simulink model "four_module_inverter_9_level_MCI"  (R2025a)
settings: Solver=VariableStepAuto  StartTime=0.0  StopTime=1  RelTol=1e-3
undefined symbols (not defined in the file): Ion, Lithium
libraries: spsIGBTDiodeLib x16, simulink x8, spsCurrentMeasurementLib x6, spsBreakerLib x4, spsBatteryLib x4, spsVoltageMeasurementLib x3, spsRMSLib x1, spsTHDLib x1, sps_lib x1
settings Model: Creator=mugun  LastModifiedBy=mugun
settings DataIOCC: SaveFormat=StructureWithTime  LoggingToFile=on

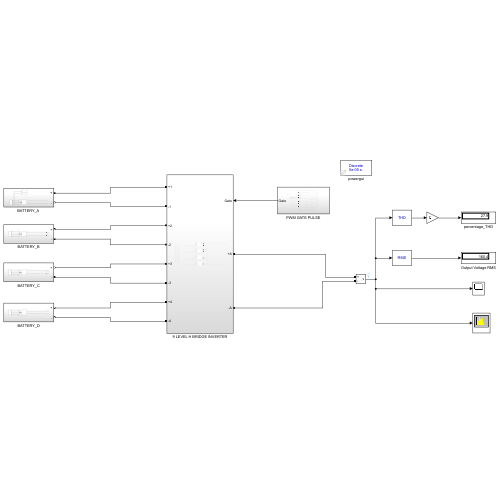
[thumbnail: Simulink's stored preview of the top-level diagram]
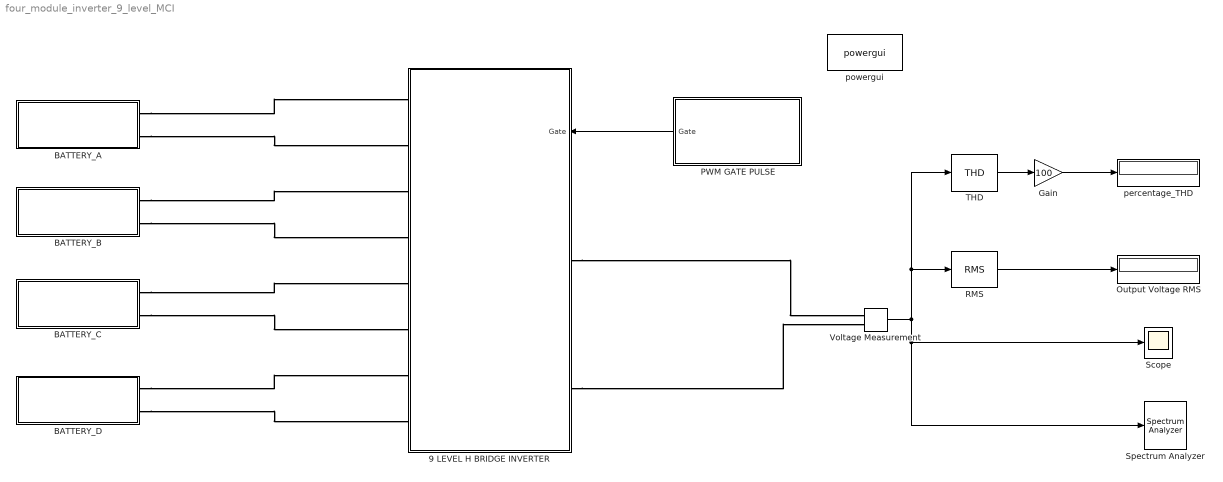
== system four_module_inverter_9_level_MCI ==
  9 LEVEL H BRIDGE INVERTER : Subsystem
      settings: PortSchema="{\"entries\":[{\"content\":{\"sides\":[{\"content\":{\"connectorIds\":[\"LConn1\",\"LConn2\",\"LConn3\",\"LConn4\",\"LConn5\",\"LConn6\",\"LConn7\",\"LConn8\"]},\"type\":\"ConnectorPlacement.EquallySpacedRectSide\",\"uuid\":\"a99ba5a4-868b-4ca9-ae89-158e30df76de\"},{\"content\":{\"connectorIds\":[\"In1\",\"RConn1\",\"RConn2\"],\"side\":\"RIGHT\"},\"type\":\"ConnectorPlacement.EquallySpacedRectSide\",\"uuid\":\"907b6b32-6b28-4f9b-aa63-058c17a50e82\"},{\"content\":{\"side\":\"TOP\"},\"type\":\"ConnectorPlacement.EquallySpacedRectSide\",\"uuid\":\"64bd340d-5502-4b77-92cb-0ed146f38aa8\"}]},\"type\":\"ConnectorPlacement.EquallySpacedConnector\",\"uuid\":\"1fa2cca1-805b-4996-9e9c-123ddddb2b33\"}],\"packageUris\":[\"http://schema.mathworks.com/mf0/Connector/R2020b\"],\"version\":\"1.0\"}"
  "BATTERY_A " : Subsystem
  BATTERY_B : Subsystem
  BATTERY_C : Subsystem
  BATTERY_D : Subsystem
  Gain : Gain  Gain=100
  Output Voltage RMS : Display
  PWM GATE PULSE : Subsystem
  RMS : spsRMSLib/RMS  TrueRMS=on  Freq=60  RMSInit=120  Ts=0
  Scope : Scope
      settings: ActiveDisplayYMinimum=-302.46098091950148  ActiveDisplayYMaximum=306.52866411781525  DataLoggingVariableName=MCI_nine
  Spectrum Analyzer : SpectrumAnalyzer  WindowPosition=[1.000000,49.000000,1536.000000,793.000000,]  ScopeFrameLocation=window  Method=Welch  PlotAsTwoSidedSpectrum=off  AveragingMethod=Exponential  MaximizeAxes=Off  YLimits=[-0.4051 87.1177]  SelectedToolstripTab=spectrumAnalyzerToolstrip.measurementsTab
  THD : spsTHDLib/THD  Freq=60  Ts=0
  Voltage Measurement : spsVoltageMeasurementLib/Voltage Measurement  PhasorSimulation=off  OutputType=Complex  PSBequivalent=0
  percentage_THD : Display
  powergui : sps_lib/powergui  Priority=1  SimulationMode=Discrete  SampleTime=50e-6  frequency=60  Iterations=50  frequencyindice=0  Pbase=100e6  ErrMax=1e-4  UnitsV=kV  UnitsW=MW  buscounter=0  FunctionMessages=off  echomessages=off  EnableUseOfTLC=off  CurrentSourceSwitches=off  DisableSnubberDevices=off  DisableRonSwitches=off  DisableVfSwitches=off  DisplayEquations=off  AutomaticDiscreteSolvers=off  SolverType=Tustin/Backward Euler (TBE)  Interpol=off  ExternalGateDelay=off  methode=off  Ts=100  x0status=blocks  SPID=on  SwTol=0  HookPort=off  NonlinearTolerance=1e-4  nMaxIteration=100  ContinueOnMaxIteration=off  RestoreLinks=warning  ResistiveCurrentMeasurement=off  Frange=[0:2:500]  Ylog=off  Xlog=on  ShowGrid=off  save=off  variable=ZData  structure=0  ZoomFFT=off  StartTime=0.0  cycles=1  DisplayStyle=1  fundamental=60  FreqAxis=off  MaxFrequency=1000  frequencyindicesteady=1  RmsSteady=1  display=off
  wires:
  PWM GATE PULSE/1(Gate) -> 9 LEVEL H BRIDGE INVERTER/1(Gate)
  Voltage Measurement/1 -> Scope/1, Spectrum Analyzer/1, THD/1, RMS/1
  RMS/1 -> Output Voltage RMS/1
  THD/1 -> Gain/1
  Gain/1 -> percentage_THD/1
  connections:
  BATTERY_D/LConn1 -- 9 LEVEL H BRIDGE INVERTER/LConn7
  BATTERY_C/LConn1 -- 9 LEVEL H BRIDGE INVERTER/LConn5
  BATTERY_D/LConn2 -- 9 LEVEL H BRIDGE INVERTER/LConn8
  BATTERY_C/LConn2 -- 9 LEVEL H BRIDGE INVERTER/LConn6
  BATTERY_B/LConn2 -- 9 LEVEL H BRIDGE INVERTER/LConn4
  9 LEVEL H BRIDGE INVERTER/RConn2 -- Voltage Measurement/LConn2
  "BATTERY_A "/LConn1 -- 9 LEVEL H BRIDGE INVERTER/LConn1
  "BATTERY_A "/LConn2 -- 9 LEVEL H BRIDGE INVERTER/LConn2
  BATTERY_B/LConn1 -- 9 LEVEL H BRIDGE INVERTER/LConn3
  9 LEVEL H BRIDGE INVERTER/RConn1 -- Voltage Measurement/LConn1

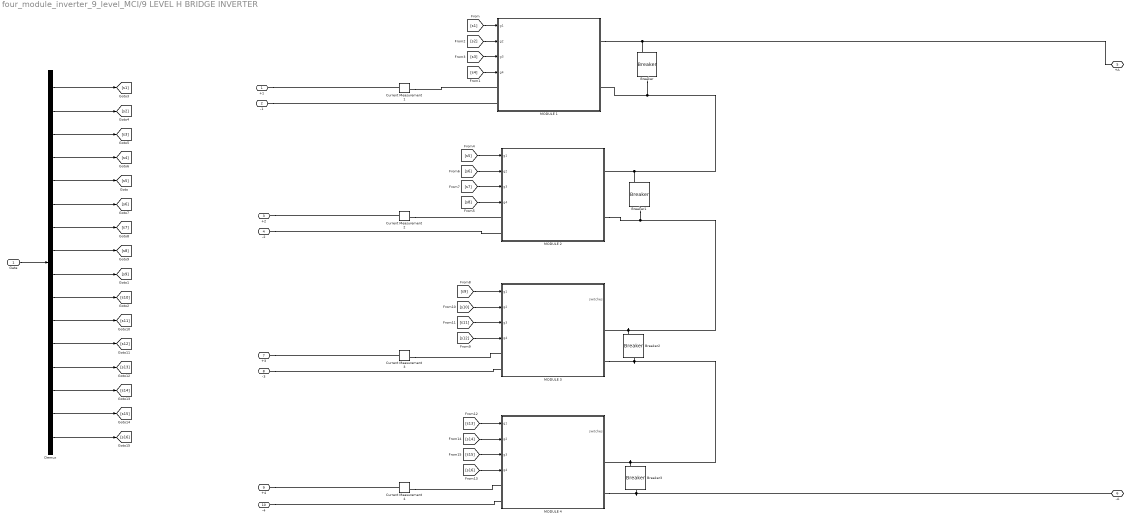
== system four_module_inverter_9_level_MCI/9 LEVEL H BRIDGE INVERTER ==
  Gate : Inport
  Breaker{,1..3} (4 alike) : spsBreakerLib/Breaker  InitialState=0  SwitchingTimes="[1/60  5/60]"  External=on  BreakerResistance=0.01  SnubberResistance=1e10  SnubberCapacitance=inf  Measurements=None  MoreParameters=on  NoBreakLoop=off
  Current Measurement{1..4} (4 alike) : spsCurrentMeasurementLib/Current Measurement  PhasorSimulation=off  OutputType=Complex  PSBequivalent=0
  Demux : Demux  Outputs=16
  MODULE 1 : Subsystem
  MODULE 2 : Subsystem
  MODULE 3 : Subsystem
  MODULE 4 : Subsystem
  +1 : PMIOPort  Side=Left
  -1 : PMIOPort  Port=2  Side=Left
  +2 : PMIOPort  Port=3  Side=Left
  -2 : PMIOPort  Port=4  Side=Left
  +A : PMIOPort  Port=5  Side=Right
  -A : PMIOPort  Port=6  Side=Right
  +3 : PMIOPort  Port=7  Side=Left
  -3 : PMIOPort  Port=8  Side=Left
  +4 : PMIOPort  Port=9  Side=Left
  -4 : PMIOPort  Port=10  Side=Left
  wires:
  Demux/1 -> [s1]
  Demux/2 -> [s2]
  Demux/3 -> [s3]
  Demux/4 -> [s4]
  Demux/5 -> [s5]
  Demux/6 -> [s6]
  Demux/7 -> [s7]
  Demux/8 -> [s8]
  Gate/1 -> Demux/1
  Demux/9 -> [s9]
  Demux/10 -> [s10]
  Demux/11 -> [s11]
  Demux/12 -> [s12]
  Demux/16 -> [s16]
  Demux/15 -> [s15]
  Demux/14 -> [s14]
  Demux/13 -> [s13]
  [s3] -> MODULE 1/3(g3)
  [s1] -> MODULE 1/1(g1)
  [s4] -> MODULE 1/4(g4)
  [s2] -> MODULE 1/2(g2)
  [s6] -> MODULE 2/2(g2)
  [s8] -> MODULE 2/4(g4)
  [s5] -> MODULE 2/1(g1)
  [s7] -> MODULE 2/3(g3)
  [s10] -> MODULE 3/2(g2)
  [s12] -> MODULE 3/4(g4)
  [s9] -> MODULE 3/1(g1)
  [s11] -> MODULE 3/3(g3)
  [s14] -> MODULE 4/2(g2)
  [s16] -> MODULE 4/4(g4)
  [s13] -> MODULE 4/1(g1)
  [s15] -> MODULE 4/3(g3)
  connections:
  +1/RConn1 -- Current Measurement1/LConn1
  Current Measurement1/RConn1 -- MODULE 1/LConn1
  -1/RConn1 -- MODULE 1/LConn2
  Current Measurement2/RConn1 -- MODULE 2/LConn1
  -2/RConn1 -- MODULE 2/LConn2
  +2/RConn1 -- Current Measurement2/LConn1
  Current Measurement3/RConn1 -- MODULE 3/LConn1
  -3/RConn1 -- MODULE 3/LConn2
  +3/RConn1 -- Current Measurement3/LConn1
  Current Measurement4/RConn1 -- MODULE 4/LConn1
  -4/RConn1 -- MODULE 4/LConn2
  +4/RConn1 -- Current Measurement4/LConn1
  Breaker/RConn1 -- MODULE 1/RConn2 -- MODULE 2/RConn1 -- Breaker1/LConn1
  Breaker2/LConn1 -- MODULE 3/RConn1 -- MODULE 2/RConn2 -- Breaker1/RConn1
  MODULE 3/RConn2 -- Breaker2/RConn1 -- MODULE 4/RConn1 -- Breaker3/LConn1
  MODULE 4/RConn2 -- Breaker3/RConn1 -- -A/RConn1
  MODULE 1/RConn1 -- Breaker/LConn1 -- +A/RConn1

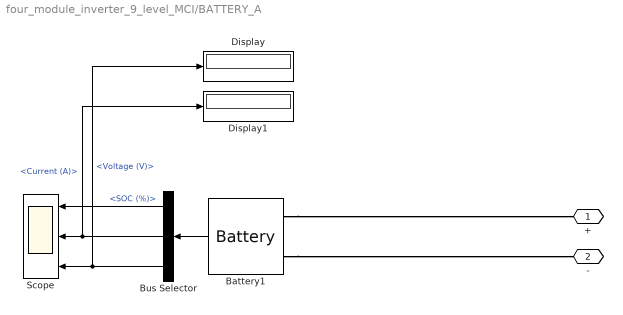
== system four_module_inverter_9_level_MCI/BATTERY_A  ==
  Battery1 : spsBatteryLib/Battery  BatType=Lithium-Ion  NomV=50  NomQ=110  SOC=80  Batt_Tr=30  PresetModel=on  MaxQ=110  MinV=37.5  FullV=58.1994  Dis_rate=47.8261  R=0.0045455  Normal_OP=99.4783  expZone="[54.0193      5.40435]"
  Bus Selector : BusSelector  OutputSignals=SOC (%),Current (A),Voltage (V)
  Display : Display
  Display1 : Display
  Scope : Scope  NumInputPorts=3
      settings: ActiveDisplayYMinimum=80.6576402320921  ActiveDisplayYMaximum=80.657640232110069
  + : PMIOPort  Side=Left
  - : PMIOPort  Port=2  Side=Left
  wires:
  Bus Selector/3 -> Display/1, Scope/3  "<Voltage (V)>"
  Battery1/1 -> Bus Selector/1
  Bus Selector/2 -> Display1/1, Scope/2  "<Current (A)>"
  Bus Selector/1 -> Scope/1  "<SOC (%)>"
  connections:
  Battery1/LConn2 -- -/RConn1
  Battery1/LConn1 -- +/RConn1

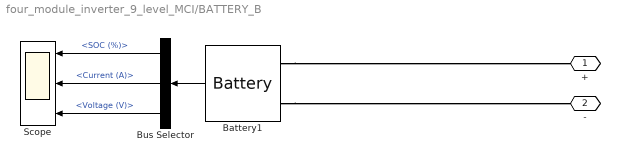
== system four_module_inverter_9_level_MCI/BATTERY_B ==
  Battery1 : spsBatteryLib/Battery  BatType=Lithium-Ion  NomV=50  NomQ=110  SOC=80  Batt_Tr=30  PresetModel=on  MaxQ=110  MinV=37.5  FullV=58.1994  Dis_rate=47.8261  R=0.0045455  Normal_OP=99.4783  expZone="[54.0193      5.40435]"
  Bus Selector : BusSelector  OutputSignals=SOC (%),Current (A),Voltage (V)
  Scope : Scope  NumInputPorts=3
      settings: ActiveDisplayYMinimum=80.6576402320921  ActiveDisplayYMaximum=80.657640232110069
  + : PMIOPort  Side=Left
  - : PMIOPort  Port=2  Side=Left
  wires:
  Bus Selector/3 -> Scope/3  "<Voltage (V)>"
  Battery1/1 -> Bus Selector/1
  Bus Selector/2 -> Scope/2  "<Current (A)>"
  Bus Selector/1 -> Scope/1  "<SOC (%)>"
  connections:
  Battery1/LConn2 -- -/RConn1
  Battery1/LConn1 -- +/RConn1

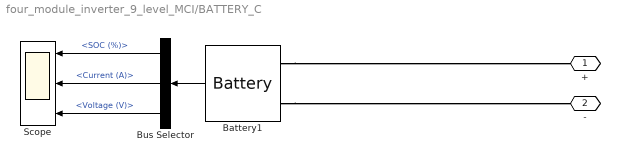
== system four_module_inverter_9_level_MCI/BATTERY_C ==
  Battery1 : spsBatteryLib/Battery  BatType=Lithium-Ion  NomV=50  NomQ=110  SOC=80  Batt_Tr=30  PresetModel=on  MaxQ=110  MinV=37.5  FullV=58.1994  Dis_rate=47.8261  R=0.0045455  Normal_OP=99.4783  expZone="[54.0193      5.40435]"
  Bus Selector : BusSelector  OutputSignals=SOC (%),Current (A),Voltage (V)
  Scope : Scope  NumInputPorts=3
      settings: ActiveDisplayYMinimum=80.6576402320921  ActiveDisplayYMaximum=80.657640232110069
  + : PMIOPort  Side=Left
  - : PMIOPort  Port=2  Side=Left
  wires:
  Bus Selector/3 -> Scope/3  "<Voltage (V)>"
  Battery1/1 -> Bus Selector/1
  Bus Selector/2 -> Scope/2  "<Current (A)>"
  Bus Selector/1 -> Scope/1  "<SOC (%)>"
  connections:
  Battery1/LConn2 -- -/RConn1
  Battery1/LConn1 -- +/RConn1

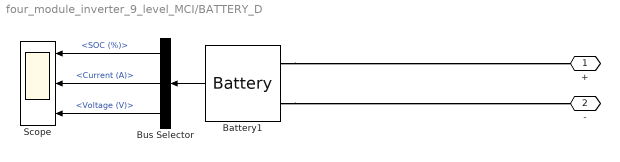
== system four_module_inverter_9_level_MCI/BATTERY_D ==
  Battery1 : spsBatteryLib/Battery  BatType=Lithium-Ion  NomV=50  NomQ=110  SOC=80  Batt_Tr=30  PresetModel=on  MaxQ=110  MinV=37.5  FullV=58.1994  Dis_rate=47.8261  R=0.0045455  Normal_OP=99.4783  expZone="[54.0193      5.40435]"
  Bus Selector : BusSelector  OutputSignals=SOC (%),Current (A),Voltage (V)
  Scope : Scope  NumInputPorts=3
      settings: ActiveDisplayYMinimum=80.6576402320921  ActiveDisplayYMaximum=80.657640232110069
  + : PMIOPort  Side=Left
  - : PMIOPort  Port=2  Side=Left
  wires:
  Bus Selector/3 -> Scope/3  "<Voltage (V)>"
  Battery1/1 -> Bus Selector/1
  Bus Selector/2 -> Scope/2  "<Current (A)>"
  Bus Selector/1 -> Scope/1  "<SOC (%)>"
  connections:
  Battery1/LConn2 -- -/RConn1
  Battery1/LConn1 -- +/RConn1

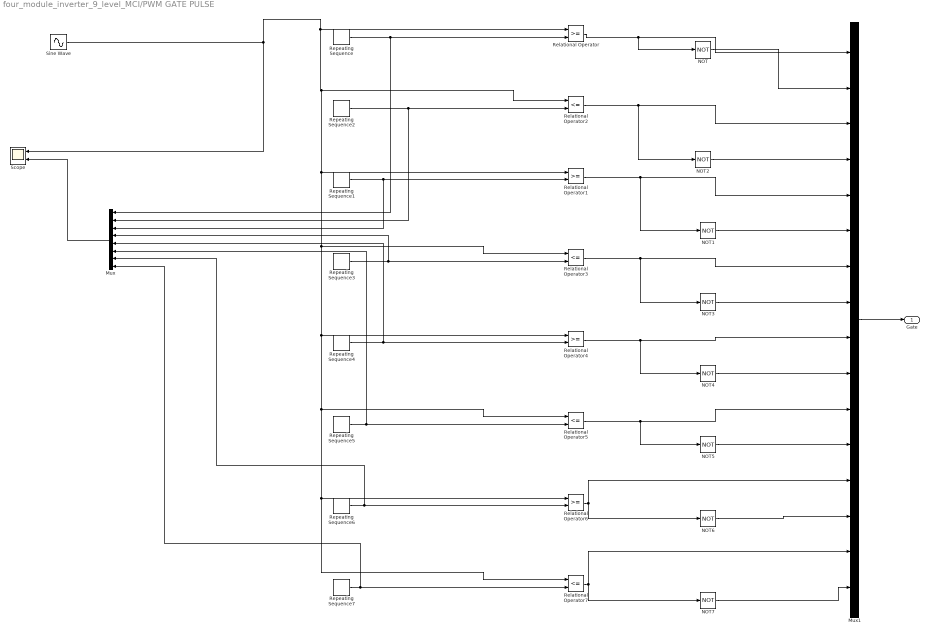
== system four_module_inverter_9_level_MCI/PWM GATE PULSE ==
  Mux : Mux  Inputs=8
  Mux1 : Mux  Inputs=16
  NOT{,1..7} (8 alike) : Logic  Operator=NOT  IconShape=distinctive  AllPortsSameDT=off  OutDataTypeStr=boolean
  Relational Operator{,1,4,6} (4 alike) : RelationalOperator  OutDataTypeStr=boolean  RndMeth=Simplest  InputSameDT=off
  Relational Operator{2..3,5,7} (4 alike) : RelationalOperator  Operator=<=  OutDataTypeStr=boolean  RndMeth=Simplest  InputSameDT=off
  Repeating Sequence : simulink/Sources/Repeating Sequence  rep_seq_t=([0 0.5 1])/1000  rep_seq_y=[3 4 3]
  Repeating Sequence1 : simulink/Sources/Repeating Sequence  rep_seq_t=([0 0.5 1])/1000  rep_seq_y=[1 2 1]
  Repeating Sequence2 : simulink/Sources/Repeating Sequence  rep_seq_t=([0 0.5 1])/1000  rep_seq_y=[2 3 2]
  Repeating Sequence3 : simulink/Sources/Repeating Sequence  rep_seq_t=([0 0.5 1])/1000  rep_seq_y=[0 1 0]
  Repeating Sequence4 : simulink/Sources/Repeating Sequence  rep_seq_t=([0 0.5 1])/1000  rep_seq_y=[-1 0 -1]
  Repeating Sequence5 : simulink/Sources/Repeating Sequence  rep_seq_t=([0 0.5 1])/1000  rep_seq_y=[-2 -1 -2]
  Repeating Sequence6 : simulink/Sources/Repeating Sequence  rep_seq_t=([0 0.5 1])/1000  rep_seq_y=[-3 -2 -3]
  Repeating Sequence7 : simulink/Sources/Repeating Sequence  rep_seq_t=([0 0.5 1])/1000  rep_seq_y=[-4 -3 -4]
  Scope : Scope  NumInputPorts=2
      settings: ActiveDisplayYMinimum=-5  ActiveDisplayYMaximum=5
  Sine Wave : Sin  Amplitude=4  Frequency=2*pi*50  SampleTime=0  VectorParams1D=off
  Gate : Outport
  wires:
  Repeating Sequence/1 -> Mux/1, Relational Operator/2
  Relational Operator/1 -> Mux1/1, NOT/1
  Repeating Sequence1/1 -> Mux/3, Relational Operator1/2
  Relational Operator1/1 -> NOT1/1, Mux1/5
  NOT/1 -> Mux1/2
  NOT1/1 -> Mux1/6
  NOT2/1 -> Mux1/4
  Repeating Sequence2/1 -> Mux/2, Relational Operator2/2
  Relational Operator2/1 -> NOT2/1, Mux1/3
  Relational Operator3/1 -> Mux1/7, NOT3/1
  Repeating Sequence3/1 -> Mux/4, Relational Operator3/2
  NOT3/1 -> Mux1/8
  Mux/1 -> Scope/2
  NOT5/1 -> Mux1/12
  Relational Operator5/1 -> Mux1/11, NOT5/1
  Repeating Sequence5/1 -> Relational Operator5/2, Mux/6
  Repeating Sequence4/1 -> Mux/5, Relational Operator4/2
  Relational Operator4/1 -> Mux1/9, NOT4/1
  NOT4/1 -> Mux1/10
  Mux1/1 -> Gate/1
  Sine Wave/1 -> Relational Operator2/1, Relational Operator7/1, Relational Operator6/1, Relational Operator5/1, Relational Operator4/1, Relational Operator3/1, Relational Operator1/1, Relational Operator/1, Scope/1
  NOT6/1 -> Mux1/14
  Repeating Sequence6/1 -> Mux/7, Relational Operator6/2
  Repeating Sequence7/1 -> Mux/8, Relational Operator7/2
  Relational Operator7/1 -> Mux1/15, NOT7/1
  Relational Operator6/1 -> Mux1/13, NOT6/1
  NOT7/1 -> Mux1/16

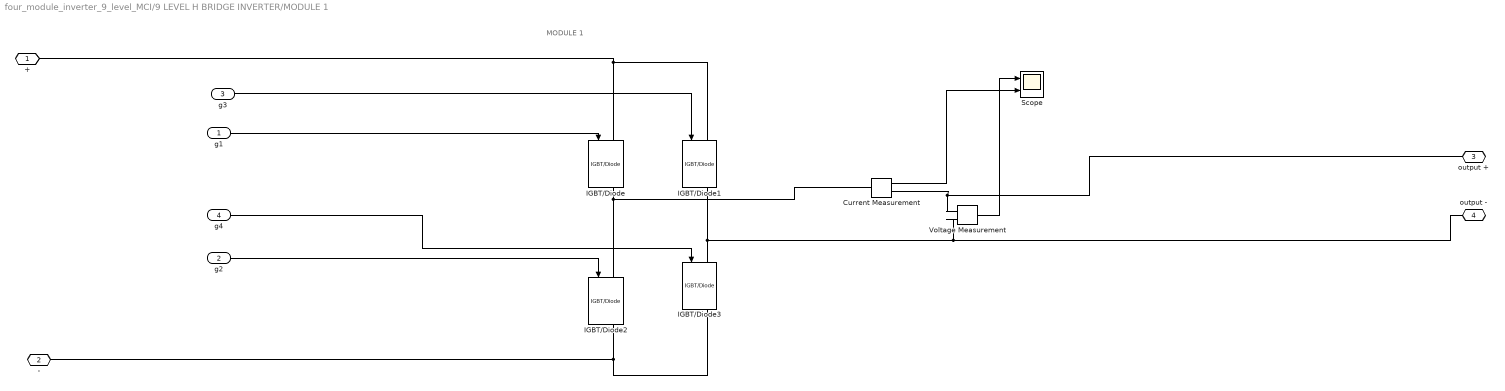
== system four_module_inverter_9_level_MCI/9 LEVEL H BRIDGE INVERTER/MODULE 1 ==
  note: MODULE 1
  g1 : Inport
  g2 : Inport  Port=2
  g3 : Inport  Port=3
  g4 : Inport  Port=4
  Current Measurement : spsCurrentMeasurementLib/Current Measurement  PhasorSimulation=off  OutputType=Complex  PSBequivalent=0
  IGBT/Diode{,1..3} (4 alike) : spsIGBTDiodeLib/IGBT//Diode  Ron=1e-3  Rs=1e5  Cs=inf  Measurements=on
  Scope : Scope  NumInputPorts=2
      settings: ActiveDisplayYMinimum=-67.656399857092211  ActiveDisplayYMaximum=67.656345987022974  DataLoggingVariableName=ScopeData2
  Voltage Measurement : spsVoltageMeasurementLib/Voltage Measurement  PhasorSimulation=off  OutputType=Complex  PSBequivalent=0
  + : PMIOPort  Side=Left
  - : PMIOPort  Port=2  Side=Left
  output + : PMIOPort  Port=3  Side=Right
  output - : PMIOPort  Port=4  Side=Right
  wires:
  g3/1 -> IGBT/Diode1/1
  g1/1 -> IGBT/Diode/1
  g2/1 -> IGBT/Diode2/1
  g4/1 -> IGBT/Diode3/1
  Voltage Measurement/1 -> Scope/1
  Current Measurement/1 -> Scope/2
  connections:
  IGBT/Diode/RConn1 -- IGBT/Diode2/LConn1 -- Current Measurement/LConn1
  IGBT/Diode1/RConn1 -- IGBT/Diode3/LConn1 -- Voltage Measurement/LConn2 -- output -/RConn1
  IGBT/Diode3/RConn1 -- -/RConn1 -- IGBT/Diode2/RConn1
  IGBT/Diode/LConn1 -- +/RConn1 -- IGBT/Diode1/LConn1
  Voltage Measurement/LConn1 -- Current Measurement/RConn1 -- output +/RConn1

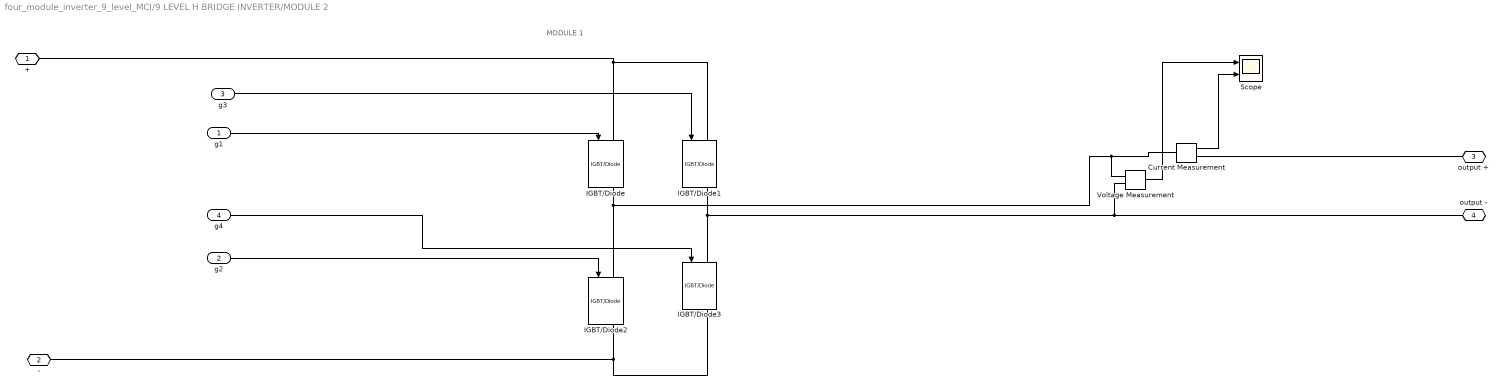
== system four_module_inverter_9_level_MCI/9 LEVEL H BRIDGE INVERTER/MODULE 2 ==
  note: MODULE 1
  g1 : Inport
  g2 : Inport  Port=2
  g3 : Inport  Port=3
  g4 : Inport  Port=4
  Current Measurement : spsCurrentMeasurementLib/Current Measurement  PhasorSimulation=off  OutputType=Complex  PSBequivalent=0
  IGBT/Diode{,1..3} (4 alike) : spsIGBTDiodeLib/IGBT//Diode  Ron=1e-3  Rs=1e5  Cs=inf  Measurements=on
  Scope : Scope  NumInputPorts=2
      settings: ActiveDisplayYMinimum=-68.11449112775864  ActiveDisplayYMaximum=67.198291734216028  DataLoggingVariableName=ScopeData3
  Voltage Measurement : spsVoltageMeasurementLib/Voltage Measurement  PhasorSimulation=off  OutputType=Complex  PSBequivalent=0
  + : PMIOPort  Side=Left
  - : PMIOPort  Port=2  Side=Left
  output + : PMIOPort  Port=3  Side=Right
  output - : PMIOPort  Port=4  Side=Right
  wires:
  g3/1 -> IGBT/Diode1/1
  g1/1 -> IGBT/Diode/1
  g2/1 -> IGBT/Diode2/1
  g4/1 -> IGBT/Diode3/1
  Voltage Measurement/1 -> Scope/1
  Current Measurement/1 -> Scope/2
  connections:
  IGBT/Diode/RConn1 -- Voltage Measurement/LConn1 -- Current Measurement/LConn1 -- IGBT/Diode2/LConn1
  IGBT/Diode1/RConn1 -- Voltage Measurement/LConn2 -- output -/RConn1 -- IGBT/Diode3/LConn1
  IGBT/Diode3/RConn1 -- IGBT/Diode2/RConn1 -- -/RConn1
  IGBT/Diode/LConn1 -- IGBT/Diode1/LConn1 -- +/RConn1
  Current Measurement/RConn1 -- output +/RConn1

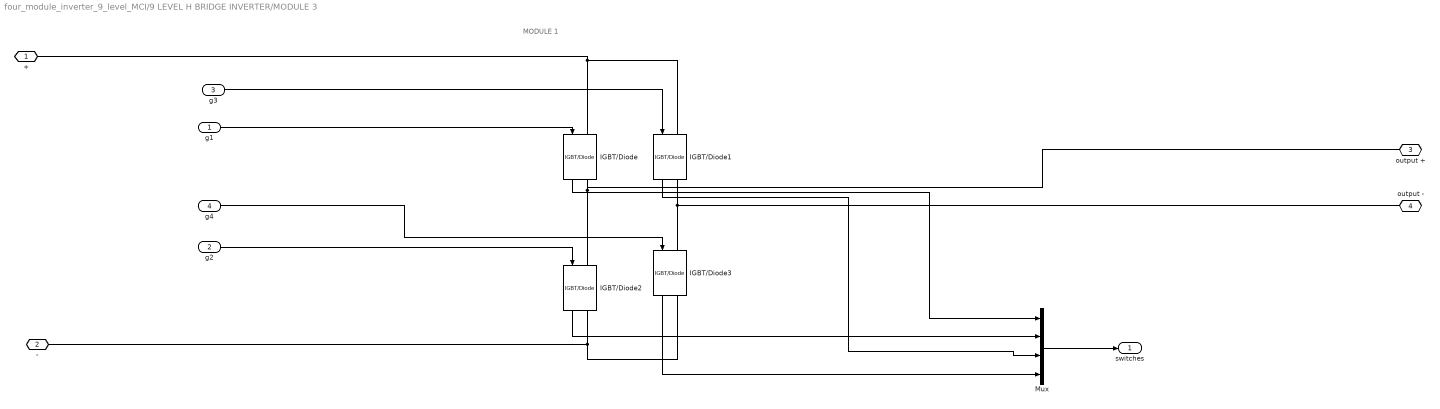
== system four_module_inverter_9_level_MCI/9 LEVEL H BRIDGE INVERTER/MODULE 3 ==
  note: MODULE 1
  g1 : Inport
  g2 : Inport  Port=2
  g3 : Inport  Port=3
  g4 : Inport  Port=4
  IGBT/Diode{,1..3} (4 alike) : spsIGBTDiodeLib/IGBT//Diode  Ron=1e-3  Rs=1e5  Cs=inf  Measurements=on
  Mux : Mux
  + : PMIOPort  Side=Left
  - : PMIOPort  Port=2  Side=Left
  output + : PMIOPort  Port=3  Side=Right
  output - : PMIOPort  Port=4  Side=Right
  switches : Outport
  wires:
  g3/1 -> IGBT/Diode1/1
  g1/1 -> IGBT/Diode/1
  IGBT/Diode2/1 -> Mux/2
  IGBT/Diode3/1 -> Mux/4
  g2/1 -> IGBT/Diode2/1
  g4/1 -> IGBT/Diode3/1
  IGBT/Diode/1 -> Mux/1
  IGBT/Diode1/1 -> Mux/3
  Mux/1 -> switches/1
  connections:
  IGBT/Diode/RConn1 -- output +/RConn1 -- IGBT/Diode2/LConn1
  IGBT/Diode1/RConn1 -- output -/RConn1 -- IGBT/Diode3/LConn1
  IGBT/Diode3/RConn1 -- IGBT/Diode2/RConn1 -- -/RConn1
  IGBT/Diode/LConn1 -- IGBT/Diode1/LConn1 -- +/RConn1

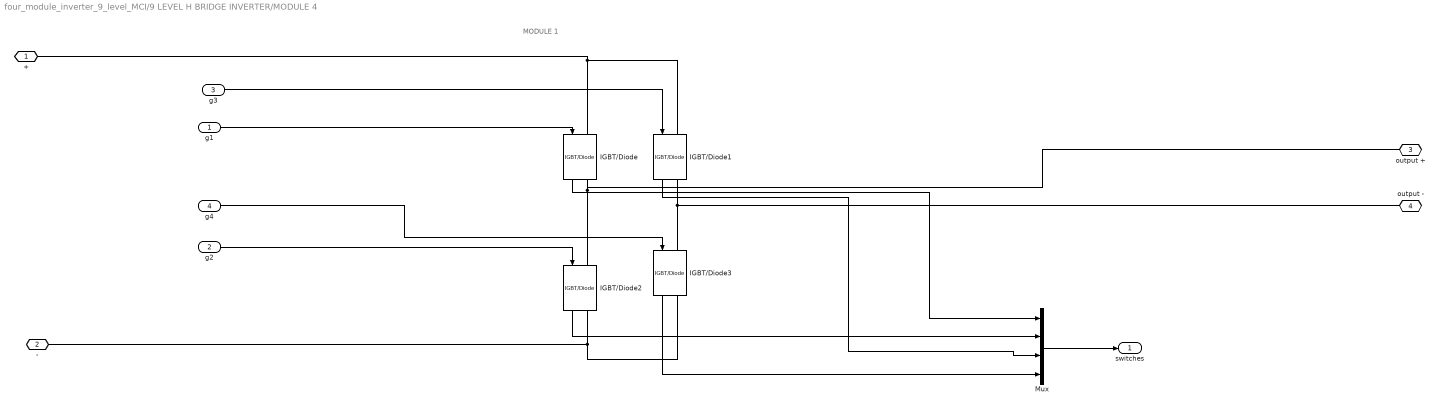
== system four_module_inverter_9_level_MCI/9 LEVEL H BRIDGE INVERTER/MODULE 4 ==
  note: MODULE 1
  g1 : Inport
  g2 : Inport  Port=2
  g3 : Inport  Port=3
  g4 : Inport  Port=4
  IGBT/Diode{,1..3} (4 alike) : spsIGBTDiodeLib/IGBT//Diode  Ron=1e-3  Rs=1e5  Cs=inf  Measurements=on
  Mux : Mux
  + : PMIOPort  Side=Left
  - : PMIOPort  Port=2  Side=Left
  output + : PMIOPort  Port=3  Side=Right
  output - : PMIOPort  Port=4  Side=Right
  switches : Outport
  wires:
  g3/1 -> IGBT/Diode1/1
  g1/1 -> IGBT/Diode/1
  IGBT/Diode2/1 -> Mux/2
  IGBT/Diode3/1 -> Mux/4
  g2/1 -> IGBT/Diode2/1
  g4/1 -> IGBT/Diode3/1
  IGBT/Diode/1 -> Mux/1
  IGBT/Diode1/1 -> Mux/3
  Mux/1 -> switches/1
  connections:
  IGBT/Diode/RConn1 -- output +/RConn1 -- IGBT/Diode2/LConn1
  IGBT/Diode1/RConn1 -- output -/RConn1 -- IGBT/Diode3/LConn1
  IGBT/Diode3/RConn1 -- IGBT/Diode2/RConn1 -- -/RConn1
  IGBT/Diode/LConn1 -- IGBT/Diode1/LConn1 -- +/RConn1
